simulink model "block04"  (R2019a)
settings: Solver=VariableStepAuto  StartTime=0.0  StopTime=10.0  RelTol=1e-3
settings Model: Creator=b1991  LastModifiedBy=b1991
settings DataIOCC: LoadExternalInput=on

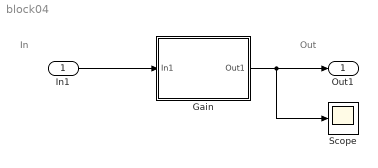
== system block04 ==
  note: Out
  note: In
  In1 : Inport
  Gain : Subsystem
  Scope : Scope
  Out1 : Outport
  wires:
  In1/1 -> Gain/1(In1)
  Gain/1(Out1) -> Scope/1, Out1/1

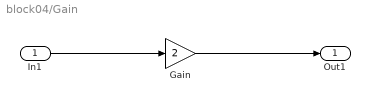
== system block04/Gain ==
  In1 : Inport
  Gain : Gain  Gain=2
  Out1 : Outport
  wires:
  Gain/1 -> Out1/1
  In1/1 -> Gain/1
